simulink library "Go_Kart_Library"  (R2018b)
settings: Solver=VariableStepAuto  StartTime=0.0  StopTime=10.0  RelTol=1e-3
settings Model: Creator=hanso  LastModifiedBy=hanso

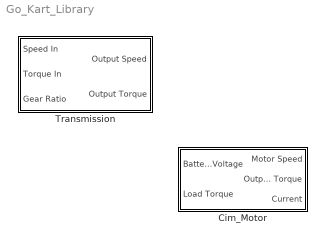
== system Go_Kart_Library ==
  Cim_Motor : Subsystem
  Transmission : Subsystem

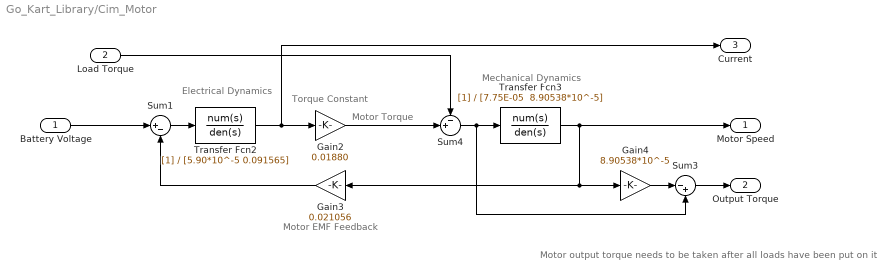
== system Go_Kart_Library/Cim_Motor ==
  note: Motor EMF Feedback
  note: Mechanical Dynamics
  note: Motor output torque needs to be taken after all loads have been put on it
  note: Motor Torque
  note: Torque Constant
  note: Electrical Dynamics
  Battery Voltage : Inport
  Load Torque : Inport  Port=2
  Gain2 : Gain  Gain=0.01880
  Gain3 : Gain  Gain=0.021056
  Gain4 : Gain  Gain=8.90538*10^-5
  Sum1 : Sum  Inputs=|+-
  Sum3 : Sum  Inputs=|-+
  Sum4 : Sum  Inputs=-+|
  Transfer Fcn2 : TransferFcn  Denominator=[5.90*10^-5 0.091565]
  Transfer Fcn3 : TransferFcn  Denominator=|
      | [7.75E-05
      |  8.90538*10^-5]
  Motor Speed : Outport
  Output Torque : Outport  Port=2
  Current : Outport  Port=3
  wires:
  Sum3/1 -> Output Torque/1
  Gain4/1 -> Sum3/1
  Transfer Fcn2/1 -> Current/1, Gain2/1
  Gain2/1 -> Sum4/2
  Sum4/1 -> Sum3/2, Transfer Fcn3/1
  Gain3/1 -> Sum1/2
  Transfer Fcn3/1 -> Motor Speed/1, Gain4/1, Gain3/1
  Sum1/1 -> Transfer Fcn2/1
  Battery Voltage/1 -> Sum1/1
  Load Torque/1 -> Sum4/1

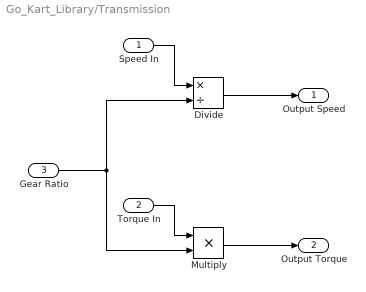
== system Go_Kart_Library/Transmission ==
  "Speed In " : Inport
  Torque In : Inport  Port=2
  Gear Ratio : Inport  Port=3
  Divide : Product  Inputs=*/
  Multiply : Product
  "Output Speed " : Outport
  "Output Torque " : Outport  Port=2
  wires:
  Torque In/1 -> Multiply/1
  Multiply/1 -> "Output Torque "/1
  "Speed In "/1 -> Divide/1
  Divide/1 -> "Output Speed "/1
  Gear Ratio/1 -> Divide/2, Multiply/2
